simulink model "Internal_Model_Control__Ramp_Input"  (R2020a)
settings: Solver=FixedStepAuto  StartTime=0.0  StopTime=2  FixedStep=0.01  RelTol=1e-3
undefined symbols (not defined in the file): A, B, C, D, K_1, K_2, K_3, L, ramp_ini_value, ramp_slope
libraries: simulink x1
settings Model: Creator=sabir  LastModifiedBy=sabir

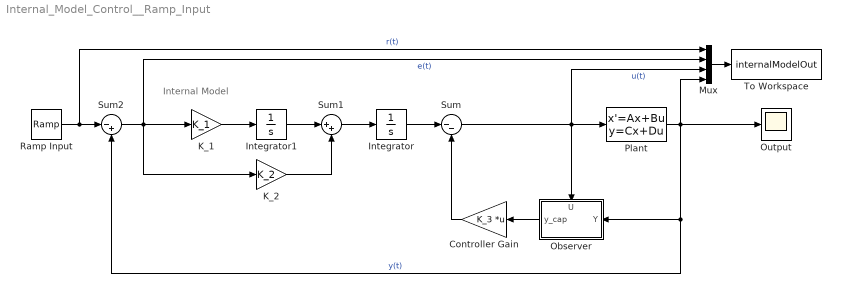
== system Internal_Model_Control__Ramp_Input ==
  note: Internal Model
  Controller Gain : Gain  Gain=K_3  Multiplication=Matrix(K*u)
  Integrator : Integrator
  Integrator1 : Integrator
  K_1 : Gain  Gain=K_1
  K_2 : Gain  Gain=K_2
  Mux : Mux
  Observer : Subsystem
      settings: PortSchema="{\"entries\":[{\"content\":{\"sides\":[{\"content\":{\"connectorIds\":[\"In1\"]},\"type\":\"ConnectorPlacement.EquallySpacedRectSide\",\"uuid\":\"a807c3ae-d956-4e18-b162-a199426d84e0\"},{\"content\":{\"connectorIds\":[\"Out1\"],\"side\":\"RIGHT\"},\"type\":\"ConnectorPlacement.EquallySpacedRectSide\",\"uuid\":\"d729827f-7b13-4043-b997-98b02c8fb4f1\"},{\"content\":{\"connectorIds\":[\"In2\"],\"side\":\"TOP\"},\"type\":\"ConnectorPlacement.EquallySpacedRectSide\",\"uuid\":\"48e72105-59dd-4ac7-a9f6-5fa3776798cb\"}]},\"type\":\"ConnectorPlacement.EquallySpacedConnector\",\"uuid\":\"e02df8ec-c895-4bcb-ab89-5fc21fc4f752\"}],\"packageUris\":[\"http://schema.mathworks.com/mf0/Connector/19700101\"],\"version\":\"1.0\"}"
  Output : Scope
  Plant : StateSpace  A=A  B=B  C=C  D=D  InitialCondition=0
  Ramp Input : simulink/Sources/Ramp  slope=ramp_slope  start=ramp_start  InitialOutput=ramp_ini_value
  Sum : Sum  Inputs=|--
  Sum1 : Sum  Inputs=|++
  Sum2 : Sum  Inputs=|-+
  To Workspace : ToWorkspace  VariableName=internalModelOut  SampleTime=-1
  wires:
  Observer/1(y_cap) -> Controller Gain/1
  Controller Gain/1 -> Sum/2
  Sum/1 -> Mux/3, Observer/2(U), Plant/1  "u(t)"
  Mux/1 -> To Workspace/1
  Plant/1 -> Mux/4, Output/1, Observer/1(Y), Sum2/2  "y(t)"
  Integrator/1 -> Sum/1
  K_2/1 -> Sum1/2
  K_1/1 -> Integrator1/1
  Integrator1/1 -> Sum1/1
  Sum1/1 -> Integrator/1
  Sum2/1 -> K_1/1, K_2/1, Mux/2  "e(t)"
  Ramp Input/1 -> Mux/1, Sum2/1  "r(t)"

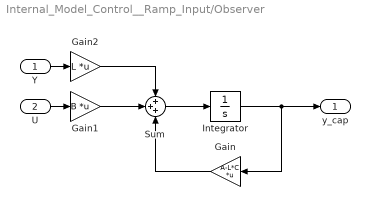
== system Internal_Model_Control__Ramp_Input/Observer ==
  Y : Inport
  U : Inport  Port=2
  Gain : Gain  Gain=A-L*C  Multiplication=Matrix(K*u)
  Gain1 : Gain  Gain=B  Multiplication=Matrix(K*u)
  Gain2 : Gain  Gain=L  Multiplication=Matrix(K*u)
  Integrator : Integrator
  Sum : Sum  Inputs=+++
  y_cap : Outport
  wires:
  Gain1/1 -> Sum/2
  Integrator/1 -> y_cap/1, Gain/1
  Gain/1 -> Sum/3
  Sum/1 -> Integrator/1
  U/1 -> Gain1/1
  Y/1 -> Gain2/1
  Gain2/1 -> Sum/1
